simulink model "Frequency_Estimator"  (R2023a)
settings: Solver=VariableStepAuto  StartTime=0.0  StopTime=128e-5  RelTol=1e-3
undefined symbols (not defined in the file or in its folder): dfilt, Radix
libraries: dspobslib x2, commchan3 x1, dspxfrm3 x1, simulink x1
settings Model: Creator=Asus  LastModifiedBy=Asus

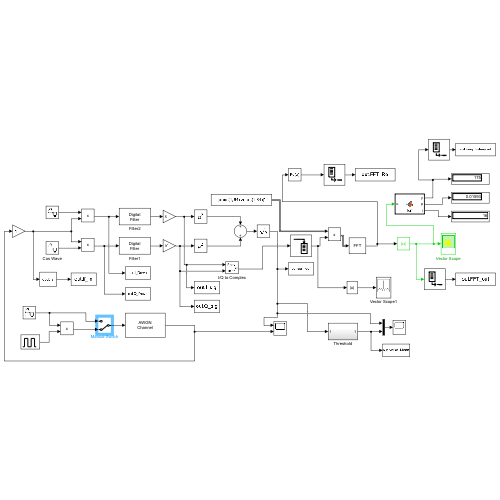
[thumbnail: Simulink's stored preview of the top-level diagram]
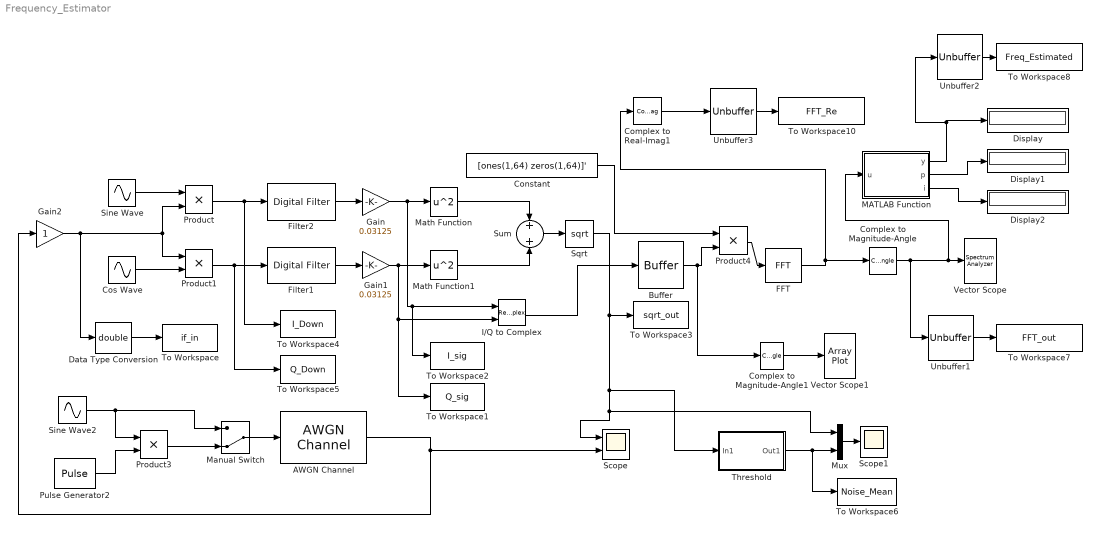
== system Frequency_Estimator ==
  AWGN Channel : commchan3/AWGN Channel  LegacyMode=on  NoiseMethod="Signal to noise ratio  (SNR)"  noiseMode="Signal to noise ratio  (SNR)"  EbNo=10  EsNo=10  SNR=10  BitsPerSymbol=1  SignalPower=0.125  SamplesPerSymbol=1  SymbolPeriod=1  VarianceSource=Parameter  Variance=1  RandomStream=Global stream  Seed=67  SimulateUsing=Code generation
  Buffer : Buffer  N=128  OutputFrames=off
  Complex to Magnitude-Angle : ComplexToMagnitudeAngle  Output=Magnitude
  Complex to Magnitude-Angle1 : ComplexToMagnitudeAngle  Output=Magnitude
  Complex to Real-Imag1 : ComplexToRealImag  Output=Real
  Constant : Constant  Value=[ones(1,64) zeros(1,64)]'  VectorParams1D=off  SampleTime=1/2e6  FramePeriod=1/1e6
      settings: SamplingMode=Frame based
  Cos Wave : Sin  Frequency=2*pi*32e6  Phase=pi/2  SampleTime=1/128e6
  Data Type Conversion : DataTypeConversion  OutDataTypeStr=double  SaturateOnIntegerOverflow=off  RndMeth=Floor
  Display : Display
  Display1 : Display
  Display2 : Display
  FFT : dspxfrm3/FFT  FFTImplementation=Radix-2  CompMethod=Table lookup  TableOpt=NEW  TableOptActive=Speed  BitRevOrder=off  Normalize=off  InheritFFTLength=off  FFTLength=128  WrapInput=on  roundingMode=Floor  overflowMode=off  firstCoeffMode=Specify word length  firstCoeffWordLength=14  firstCoeffFracLength=15  firstCoeffDataTypeStr=fixdt(1,14)  firstCoeffLastDataTypeStr=fixdt(1,14)  prodOutputMode=Binary point scaling  prodOutputWordLength=28  prodOutputFracLength=26  prodOutputDataTypeStr=fixdt(1,28,26)  prodOutputLastDataTypeStr=fixdt(1,28,26)  accumMode=Binary point scaling  accumWordLength=32  accumFracLength=26  accumDataTypeStr=fixdt(1,32,26)  accumLastDataTypeStr=fixdt(1,32,26)  outputMode=Binary point scaling  outputWordLength=14  outputFracLength=13  outputDataTypeStr=fixdt(1,14,13)  outputMin=[]  outputMax=[]  outputLastDataTypeStr=fixdt(1,14,13)
  Filter1 : dspobslib/Digital Filter  Tag=BlockMethodSubSystem  TypePopup=IIR (poles & zeros)  IIRFiltStruct=Direct form II  AllPoleFiltStruct=Direct form  FIRFiltStruct=Direct form  CoeffSource=Specify via dialog  NumCoeffs=round( [0.028 0.053 0.071 0.053 0.028].*2^20)/2^15  DenCoeffs=round( [1 -2.026 2.148 -1.159 0.279].*2^15)/2^15  BiQuadCoeffs=[1 0.3 0.4 1 0.1 0.2]  LatticeCoeffs=[0.2 0.4]  denIgnore=on  FiltPerSampPopup=One filter per frame  IC=0  ICnum=0  ICden=0  firstCoeffMode=Binary point scaling  firstCoeffWordLength=18  firstCoeffFracLength=15  outputMode=Binary point scaling  outputWordLength=14  outputFracLength=13  accumMode=Binary point scaling  accumWordLength=42  accumFracLength=35  prodOutputMode=Binary point scaling  prodOutputWordLength=42  prodOutputFracLength=35  memoryMode=Binary point scaling  memoryWordLength=24  memoryFracLength=20  roundingMode=Floor  overflowMode=off  ScaleValues=1  scaleValueFracLength=14  stageInFracLength=15  stageOutFracLength=15  FilterSource=Specify via dialog  dfiltObjectName=dfilt.dffir([1 2 1])
  Filter2 : dspobslib/Digital Filter  Tag=BlockMethodSubSystem  TypePopup=IIR (poles & zeros)  IIRFiltStruct=Direct form II  AllPoleFiltStruct=Direct form  FIRFiltStruct=Direct form  CoeffSource=Specify via dialog  NumCoeffs=round( [0.028 0.053 0.071 0.053 0.028].*2^20)/2^15  DenCoeffs=round( [1 -2.026 2.148 -1.159 0.279].*2^15)/2^15  BiQuadCoeffs=[1 0.3 0.4 1 0.1 0.2]  LatticeCoeffs=[0.2 0.4]  denIgnore=on  FiltPerSampPopup=One filter per frame  IC=0  ICnum=0  ICden=0  firstCoeffMode=Binary point scaling  firstCoeffWordLength=18  firstCoeffFracLength=15  outputMode=Binary point scaling  outputWordLength=14  outputFracLength=13  accumMode=Binary point scaling  accumWordLength=42  accumFracLength=35  prodOutputMode=Binary point scaling  prodOutputWordLength=42  prodOutputFracLength=35  memoryMode=Binary point scaling  memoryWordLength=24  memoryFracLength=20  roundingMode=Floor  overflowMode=off  ScaleValues=1  scaleValueFracLength=14  stageInFracLength=15  stageOutFracLength=15  FilterSource=Specify via dialog  dfiltObjectName=dfilt.dffir([1 2 1])
  Gain : Gain  Gain=0.03125
  Gain1 : Gain  Gain=0.03125
  Gain2 : Gain  OutDataTypeStr=fixdt(1,14,13)  RndMeth=Round  SaturateOnIntegerOverflow=on  SampleTime=1/128e6
  I/Q to Complex : RealImagToComplex
  MATLAB Function : MATLAB Function  TreatAsAtomicUnit=on
  Manual Switch : ManualSwitch  CurrentSetting=0
  Math Function : Math  Operator=square  SignedPower=on
  Math Function1 : Math  Operator=square  SignedPower=on
  Mux : Mux  Inputs=2
  Product : Product  RndMeth=Zero  SaturateOnIntegerOverflow=on
  Product1 : Product  RndMeth=Zero  SaturateOnIntegerOverflow=on
  Product3 : Product  RndMeth=Zero  SampleTime=1/128e6
  Product4 : Product  RndMeth=Zero
  Pulse Generator2 : DiscretePulseGenerator  PulseType=Time based  Period=20e-6  PulseWidth=4
  Scope : Scope  NumInputPorts=2
  Scope1 : Scope
  Sine Wave : Sin  Frequency=2*pi*32e6  SampleTime=1/128e6
  Sine Wave2 : Sin  Amplitude=.5  Frequency=2*pi*173.7e6  SampleTime=1/128e6
  Sqrt : Sqrt
  Sum : Sum  Inputs=+|+
  Threshold : Subsystem
  To Workspace : ToWorkspace  VariableName=if_in  SaveFormat=Timeseries  SampleTime=-1
  To Workspace1 : ToWorkspace  VariableName=Q_sig  SaveFormat=Timeseries  SampleTime=-1
  To Workspace10 : ToWorkspace  VariableName=FFT_Re  SaveFormat=Timeseries  SampleTime=-1
  To Workspace2 : ToWorkspace  VariableName=I_sig  SaveFormat=Timeseries  SampleTime=-1
  To Workspace3 : ToWorkspace  VariableName=sqrt_out  SaveFormat=Timeseries  SampleTime=-1
  To Workspace4 : ToWorkspace  VariableName=I_Down  SaveFormat=Timeseries  SampleTime=-1
  To Workspace5 : ToWorkspace  VariableName=Q_Down  SaveFormat=Timeseries  SampleTime=-1
  To Workspace6 : ToWorkspace  VariableName=Noise_Mean  SaveFormat=Timeseries  SampleTime=-1
  To Workspace7 : ToWorkspace  VariableName=FFT_out  SaveFormat=Timeseries  SampleTime=-1
  To Workspace8 : ToWorkspace  VariableName=Freq_Estimated  SaveFormat=Timeseries  SampleTime=-1
  Unbuffer1 : Unbuffer
  Unbuffer2 : Unbuffer
  Unbuffer3 : Unbuffer
  Vector Scope : SpectrumAnalyzer  WindowPosition=[488.000000,242.000000,560.000000,420.000000,]  ScopeFrameLocation=window  InputDomain=Frequency  SampleRate=1/(1)  FrequencySpan=Start and stop frequencies  StartFrequency=0  StopFrequency=128000000  InputUnits=Watts  SpectrumUnits=Watts  YLabel=Amplitude  YLimits=[-0.17351487,1.78995197]  ColorLimits=[-80 20]  ShowLegend=on  IsSourceVectorScope=on
  Vector Scope1 : ArrayPlot  WindowPosition=[1.000000,49.000000,1536.000000,793.000000,]  ScopeFrameLocation=window  PlotType=Line  XLabel=Time  YLimits=[-0.0144,0.1556]  ShowLegend=on
  wires:
  Gain1/1 -> To Workspace1/1, I/Q to Complex/2, Math Function1/1
  Manual Switch/1 -> AWGN Channel/1
  Filter1/1 -> Gain1/1
  Sine Wave/1 -> Product/1
  Filter2/1 -> Gain/1
  Data Type Conversion/1 -> To Workspace/1
  AWGN Channel/1 -> Gain2/1, Scope/2
  Product3/1 -> Manual Switch/2
  Cos Wave/1 -> Product1/2
  Gain2/1 -> Data Type Conversion/1, Product1/1, Product/2
  Sine Wave2/1 -> Manual Switch/1, Product3/1
  Pulse Generator2/1 -> Product3/2
  Product1/1 -> Filter1/1, To Workspace5/1
  Gain/1 -> To Workspace2/1, I/Q to Complex/1, Math Function/1
  Product/1 -> Filter2/1, To Workspace4/1
  Math Function/1 -> Sum/1
  Math Function1/1 -> Sum/2
  Sum/1 -> Sqrt/1
  Sqrt/1 -> To Workspace3/1, Threshold/1(In1), Mux/1, Scope/1
  FFT/1 -> Complex to Real-Imag1/1, Complex to Magnitude-Angle/1
  Complex to Real-Imag1/1 -> Unbuffer3/1
  Unbuffer3/1 -> To Workspace10/1
  I/Q to Complex/1 -> Buffer/1
  Complex to Magnitude-Angle/1 -> Unbuffer1/1, MATLAB Function/1(u), Vector Scope/1
  MATLAB Function/1(y) -> Display/1, Unbuffer2/1
  Complex to Magnitude-Angle1/1 -> Vector Scope1/1
  Threshold/1(Out1) -> To Workspace6/1, Mux/2
  Mux/1 -> Scope1/1
  Unbuffer1/1 -> To Workspace7/1
  Unbuffer2/1 -> To Workspace8/1
  MATLAB Function/2(p) -> Display1/1
  MATLAB Function/3(i) -> Display2/1
  Constant/1 -> Product4/1
  Buffer/1 -> Complex to Magnitude-Angle1/1, Product4/2
  Product4/1 -> FFT/1

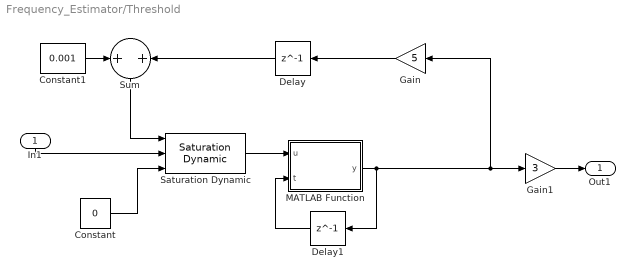
== system Frequency_Estimator/Threshold ==
  In1 : Inport
  Constant : Constant  Value=0  SampleTime=1/128e6
  Constant1 : Constant  Value=0.001  SampleTime=1/128e6
  Delay : Delay  DelayLength=1  InitialCondition=0
  Delay1 : Delay  DelayLength=1  InitialCondition=0
  Gain : Gain  Gain=5
  Gain1 : Gain  Gain=3
  MATLAB Function : MATLAB Function  TreatAsAtomicUnit=on
  Saturation Dynamic : simulink/Discontinuities/Saturation Dynamic  OutMin=[]  OutMax=[]  OutDataTypeStr=Inherit: Same as second input  OutDataType=fixdt(1, 16)  OutScaling=2^-10  DoSatur=off
  Sum : Sum  Inputs=+|+
  Out1 : Outport
  wires:
  Saturation Dynamic/1 -> MATLAB Function/1(u)
  Constant/1 -> Saturation Dynamic/3
  Sum/1 -> Saturation Dynamic/1
  Constant1/1 -> Sum/1
  Delay/1 -> Sum/2
  Gain/1 -> Delay/1
  MATLAB Function/1(y) -> Gain/1, Gain1/1, Delay1/1
  Gain1/1 -> Out1/1
  Delay1/1 -> MATLAB Function/2(t)
  In1/1 -> Saturation Dynamic/2

== matlab function Frequency_Estimator/Threshold/MATLAB Function ==
  data: u input; y output; t input
function y = fcn(u,t)

    alpha = 2^(-15);
    y = (1 - alpha) * t + alpha * u;

== matlab function Frequency_Estimator/MATLAB Function ==
  data: u input; y output; p output; i output
function [y ,p , i]= fcn(u)

[t i] = max(u);

if i == 1
    i=2;
end;

if i == 128
    i=127;
end;

a = u(i-1);
b = u(i);
c = u(i+1);

p = (a - c) / (2 * (a - 2*b + c));
y = i+p + 160 -1;
